simulink model "Lap1"  (R2021a)
settings: Solver=VariableStepAuto  StartTime=0.0  StopTime=10.0  RelTol=1e-3
settings Model: Creator=lenovo  LastModifiedBy=lenovo

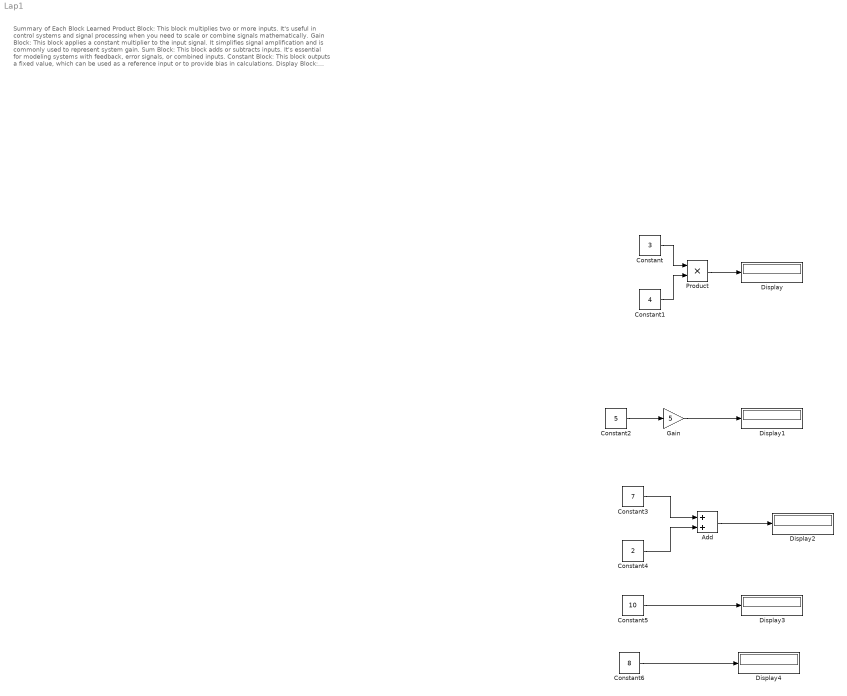
== system Lap1 ==
  note: Summary of Each Block Learned
      | Product Block:
      | This block multiplies two or more inputs. It's useful in control systems and signal processing when you need to scale or combine signals mathematically.
      | Gain Block:
      | This block applies a constant multiplier to the input signal. It simplifies signal amplification and is commonly used to represent system gain.
      | Sum Block:
      | This block adds or subtracts inputs. It's essential for modeling systems with feedback, error signals, or combined inputs.
      | Constant Block:
      | This block outputs a fixed value, which can be used as a reference input or to provide bias in calculations.
      | Display Block:
      | This block shows the value of a signal during simulation, helping to debug and monitor specific parts of the model.
      | 29. Observations and Difficulties:
      | Observations:
      | Connections between blocks are intuitive and visual, making it easier to understand system flow.
      | Simulink provides real-time feedback and easy access to simulation parameters.
      | Difficulties:
      | Initially, connecting blocks correctly and configuring parameters was a bit confusing.
      | Mislabeling of inputs in the Sum Block caused unexpected simulation results until the signs were adjusted.
      | It took some time to understand the difference between scalar and vector inputs in some blocks.
  Add : Sum
  Constant : Constant  Value=3
  Constant1 : Constant  Value=4
  Constant2 : Constant  Value=5
  Constant3 : Constant  Value=7
  Constant4 : Constant  Value=2
  Constant5 : Constant  Value=10
  Constant6 : Constant  Value=8
  Display{,1..4} (5 alike) : Display
  Gain : Gain  Gain=5
  Product : Product
  wires:
  Constant/1 -> Product/1
  Constant1/1 -> Product/2
  Product/1 -> Display/1
  Gain/1 -> Display1/1
  Constant2/1 -> Gain/1
  Constant4/1 -> Add/2
  Add/1 -> Display2/1
  Constant3/1 -> Add/1
  Constant5/1 -> Display3/1
  Constant6/1 -> Display4/1
